simulink model ""  (R2019b)
settings: Solver=VariableStepAuto  StartTime=0.0  StopTime=200  RelTol=1e-3
model workspace (MAT data in the model file):
  x2xx = 0
values from neighbouring files (symbols this model uses):
  KDspd = 0    [frequency_validation.m]
  KIspd = 0    [frequency_validation.m]
  KPspd = 20    [frequency_validation.m]
  PARSa = [ ... (first row only)    [Q_ART_par.m]
  PARSu = zeros(Nu,5)    [Q_ART_par.m]
  Q0 = zeros(Nu+2,1)    [frequency_validation.m]
  QD0 = Q0    [frequency_validation.m]
  v_ref = vconst    (= 5.55555555556)    [frequency_validation.m]
undefined symbols (not defined in the file or in its folder): axle_rate_limit, Lspd, Nspd, Tmc, Uspd
libraries: simulink x2
(part 1 of 3)
settings Model: Creator=DJW  LastModifiedBy=14668

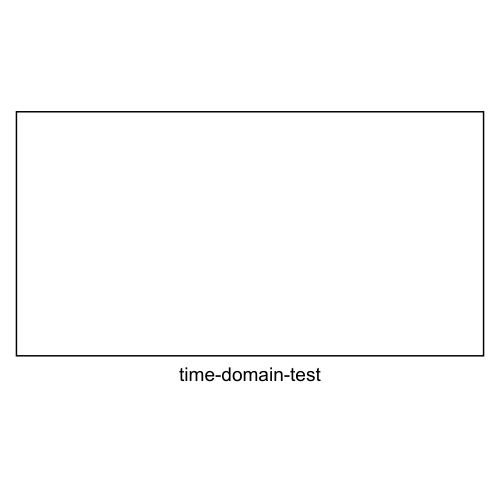
[thumbnail: Simulink's stored preview of the top-level diagram]
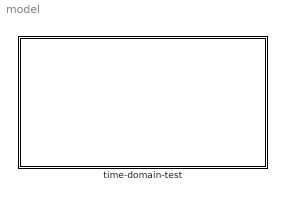
== system model ==
  time-domain-test : Subsystem

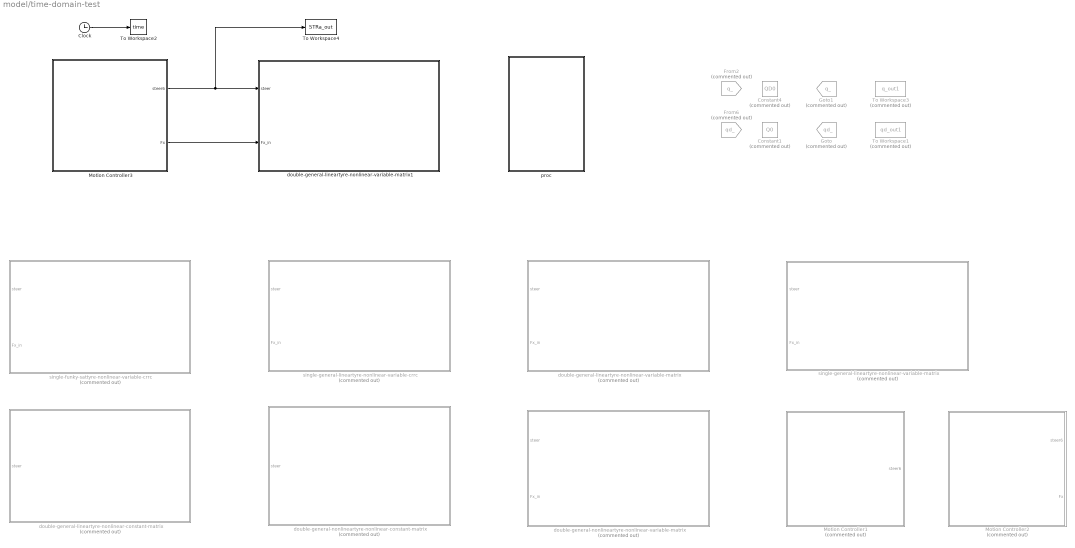
== system model/time-domain-test ==
  " Motion Controller1" : Subsystem  Commented=on  SystemSampleTime=Tmc
  " Motion Controller2" : Subsystem  Commented=on  SystemSampleTime=Tmc
  " Motion Controller3" : Subsystem  SystemSampleTime=Tmc
  Clock : Clock
  Constant1 : Constant  Commented=on  Value=Q0
  Constant4 : Constant  Commented=on  Value=QD0
  From2 : From  Commented=on  GotoTag=q_  TagVisibility=global
  From6 : From  Commented=on  GotoTag=qd_  TagVisibility=global
  Goto : Goto  Commented=on  GotoTag=qd_  TagVisibility=global
  Goto1 : Goto  Commented=on  GotoTag=q_  TagVisibility=global
  To Workspace1 : ToWorkspace  Commented=on  VariableName=qd_out1  SampleTime=-1
  To Workspace2 : ToWorkspace  VariableName=time  SampleTime=-1
  To Workspace3 : ToWorkspace  Commented=on  VariableName=q_out1  SampleTime=-1
  To Workspace4 : ToWorkspace  VariableName=STRa_out  SampleTime=-1
  double-general-lineartyre-nonlinear-constant-matrix : Subsystem  Commented=on
  double-general-lineartyre-nonlinear-variable-matrix : Subsystem  Commented=on
  double-general-lineartyre-nonlinear-variable-matrix1 : Subsystem
  double-general-nonlineartyre-nonlinear-constant-matrix : Subsystem  Commented=on
  double-general-nonlineartyre-nonlinear-variable-matrix : Subsystem  Commented=on
  proc : Subsystem
  single-funky-sattyre-nonlinear-variable-crrc : Subsystem  Commented=on
  single-general-lineartyre-nonlinear-variable-crrc : Subsystem  Commented=on
  single-general-lineartyre-nonlinear-variable-matrix : Subsystem  Commented=on
  wires:
  Clock/1 -> To Workspace2/1
  " Motion Controller3"/1(steer6) -> To Workspace4/1, double-general-lineartyre-nonlinear-variable-matrix1/1(steer)
  " Motion Controller3"/2(Fx) -> double-general-lineartyre-nonlinear-variable-matrix1/2(Fx_in)

== system model/time-domain-test/ Motion Controller1 ==
  Rate Transition6 : RateTransition
  discrete-time subsystem : Subsystem  TreatAsAtomicUnit=on  SystemSampleTime=Tmc
  steer6 : Outport
  wires:
  Rate Transition6/1 -> steer6/1
  discrete-time subsystem/1(steer) -> Rate Transition6/1

== system model/time-domain-test/ Motion Controller2 ==
  Rate Transition{3..6} (4 alike) : RateTransition
  discrete-time subsystem : Subsystem  TreatAsAtomicUnit=on  SystemSampleTime=Tmc
  steer6 : Outport
  Fx : Outport  Port=2
  wires:
  [q_] -> Rate Transition4/1
  Rate Transition5/1 -> Fx/1
  Rate Transition6/1 -> steer6/1
  [qd_] -> Rate Transition3/1
  discrete-time subsystem/1(steer) -> Rate Transition6/1
  Rate Transition4/1 -> discrete-time subsystem/1(q_in)
  Rate Transition3/1 -> discrete-time subsystem/2(qd_in)
  discrete-time subsystem/2(Fx_input) -> Rate Transition5/1

== system model/time-domain-test/ Motion Controller3 ==
  Rate Transition{3..6} (4 alike) : RateTransition
  discrete-time subsystem : Subsystem  TreatAsAtomicUnit=on  SystemSampleTime=Tmc
  steer6 : Outport
  Fx : Outport  Port=2
  wires:
  [q_] -> Rate Transition4/1
  Rate Transition5/1 -> Fx/1
  Rate Transition6/1 -> steer6/1
  [qd_] -> Rate Transition3/1
  discrete-time subsystem/1(steer) -> Rate Transition6/1
  Rate Transition4/1 -> discrete-time subsystem/1(q_in)
  Rate Transition3/1 -> discrete-time subsystem/2(qd_in)
  discrete-time subsystem/2(Fx_input) -> Rate Transition5/1

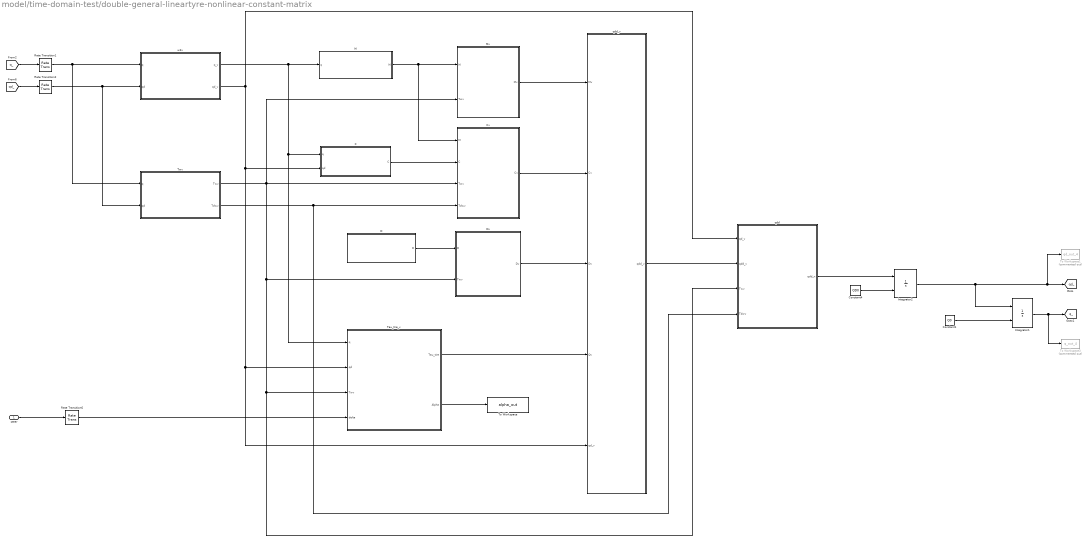
== system model/time-domain-test/double-general-lineartyre-nonlinear-constant-matrix ==
  steer : Inport
  C : MATLAB Function  TreatAsAtomicUnit=on
  Constant1 : Constant  Value=Q0
  Constant4 : Constant  Value=QD0
  Cv : MATLAB Function  TreatAsAtomicUnit=on
  D : MATLAB Function  TreatAsAtomicUnit=on
  Dv : MATLAB Function  TreatAsAtomicUnit=on
  Integrator1 : Integrator  InitialConditionSource=external  InitialCondition=Q0
  Integrator2 : Integrator  InitialConditionSource=external  InitialCondition=zeros(5,1)
  M : MATLAB Function  TreatAsAtomicUnit=on
  Mv : MATLAB Function  TreatAsAtomicUnit=on
  Rate Transition1 : RateTransition
  Rate Transition2 : RateTransition
  Rate Transition6 : RateTransition
  Tau_tire_v : MATLAB Function  TreatAsAtomicUnit=on
  To Workspace : ToWorkspace  VariableName=alpha_out  SampleTime=-1
  To Workspace1 : ToWorkspace  Commented=on  VariableName=qd_out_4  SampleTime=-1
  To Workspace3 : ToWorkspace  Commented=on  VariableName=q_out_4  SampleTime=-1
  Twv : MATLAB Function  TreatAsAtomicUnit=on
  qdd : MATLAB Function  TreatAsAtomicUnit=on
  qdd_v : MATLAB Function  TreatAsAtomicUnit=on
  w2v : MATLAB Function  TreatAsAtomicUnit=on
  tag scope: q_=global, qd_=global
  wires:
  M/1(M) -> Cv/1(M), Mv/1(M)
  [q_] -> Rate Transition1/1
  [qd_] -> Rate Transition2/1
  Twv/1(Twv) -> qdd/3(Twv), Tau_tire_v/3(Twv), Dv/2(Twv), Cv/3(Twv), Mv/2(Twv)
  C/1(C) -> Cv/2(C)
  Twv/2(Tdwv) -> qdd/4(Tdwv), Cv/4(Tdwv)
  D/1(D) -> Dv/1(D)
  steer/1 -> Rate Transition6/1
  w2v/1(q_v) -> M/1(q), Tau_tire_v/1(q), C/1(q)
  Mv/1(Mv) -> qdd_v/1(Mv)
  Dv/1(Dv) -> qdd_v/3(Dv)
  Cv/1(Cv) -> qdd_v/2(Cv)
  Tau_tire_v/1(Tau_tire) -> qdd_v/4(Qv)
  w2v/2(qd_v) -> qdd/1(qd_v), Tau_tire_v/2(qd), qdd_v/5(qd_v), C/2(qd)
  qdd_v/1(qdd_v) -> qdd/2(qdd_v)
  qdd/1(qdd_n) -> Integrator2/1
  Integrator1/1 -> To Workspace3/1, [q_]
  Integrator2/1 -> To Workspace1/1, [qd_], Integrator1/1
  Tau_tire_v/2(Alpha) -> To Workspace/1
  Constant4/1 -> Integrator2/2
  Constant1/1 -> Integrator1/2
  Rate Transition6/1 -> Tau_tire_v/4(delta)
  Rate Transition1/1 -> Twv/1(q), w2v/1(q)
  Rate Transition2/1 -> Twv/2(qd), w2v/2(qd)

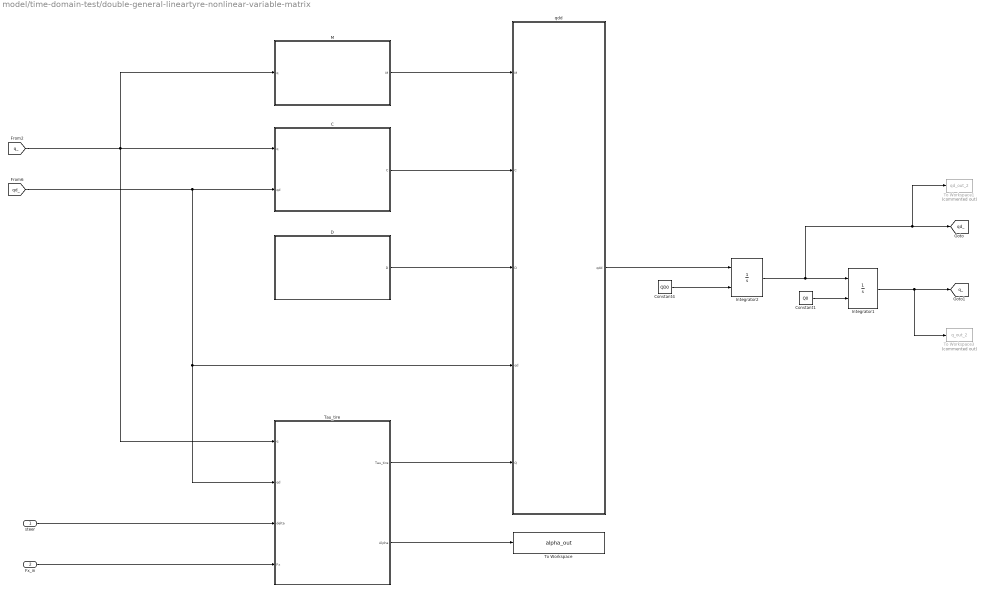
== system model/time-domain-test/double-general-lineartyre-nonlinear-variable-matrix ==
  steer : Inport
  Fx_in : Inport  Port=2
  C : MATLAB Function  TreatAsAtomicUnit=on
  Constant1 : Constant  Value=Q0
  Constant4 : Constant  Value=QD0
  D : MATLAB Function  TreatAsAtomicUnit=on
  Integrator1 : Integrator  InitialConditionSource=external  InitialCondition=Q0
  Integrator2 : Integrator  InitialConditionSource=external  InitialCondition=zeros(5,1)
  M : MATLAB Function  TreatAsAtomicUnit=on
  Tau_tire : MATLAB Function  TreatAsAtomicUnit=on
  To Workspace : ToWorkspace  VariableName=alpha_out  SampleTime=-1
  To Workspace1 : ToWorkspace  Commented=on  VariableName=qd_out_2  SampleTime=-1
  To Workspace3 : ToWorkspace  Commented=on  VariableName=q_out_2  SampleTime=-1
  qdd : MATLAB Function  TreatAsAtomicUnit=on
  tag scope: q_=global, qd_=global
  wires:
  Integrator1/1 -> To Workspace3/1, [q_]
  Fx_in/1 -> Tau_tire/4(Fx)
  [q_] -> Tau_tire/1(q), M/1(q), C/1(q)
  [qd_] -> Tau_tire/2(qd), qdd/4(qd), C/2(qd)
  steer/1 -> Tau_tire/3(delta)
  Tau_tire/2(Alpha) -> To Workspace/1
  qdd/1(qdd) -> Integrator2/1
  Integrator2/1 -> To Workspace1/1, [qd_], Integrator1/1
  M/1(M) -> qdd/1(M)
  C/1(C) -> qdd/2(C)
  Tau_tire/1(Tau_tire) -> qdd/5(Q)
  D/1(D) -> qdd/3(D)
  Constant4/1 -> Integrator2/2
  Constant1/1 -> Integrator1/2

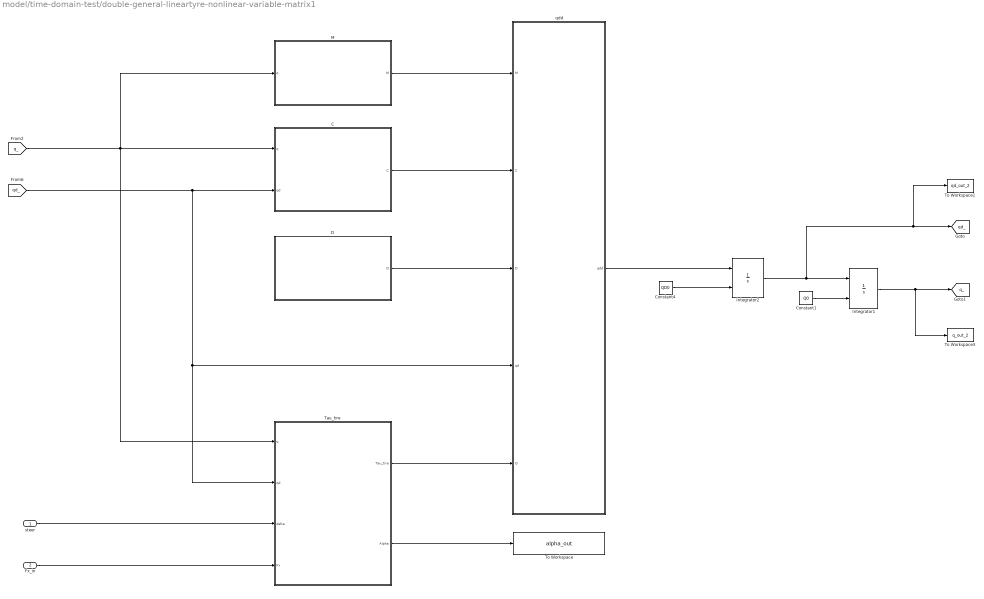
== system model/time-domain-test/double-general-lineartyre-nonlinear-variable-matrix1 ==
  steer : Inport
  Fx_in : Inport  Port=2
  C : MATLAB Function  TreatAsAtomicUnit=on
  Constant1 : Constant  Value=Q0
  Constant4 : Constant  Value=QD0
  D : MATLAB Function  TreatAsAtomicUnit=on
  Integrator1 : Integrator  InitialConditionSource=external  InitialCondition=Q0
  Integrator2 : Integrator  InitialConditionSource=external  InitialCondition=zeros(5,1)
  M : MATLAB Function  TreatAsAtomicUnit=on
  Tau_tire : MATLAB Function  TreatAsAtomicUnit=on
  To Workspace : ToWorkspace  VariableName=alpha_out  SampleTime=-1
  To Workspace1 : ToWorkspace  VariableName=qd_out_2  SampleTime=-1
  To Workspace3 : ToWorkspace  VariableName=q_out_2  SampleTime=-1
  qdd : MATLAB Function  TreatAsAtomicUnit=on
  tag scope: q_=global, qd_=global
  wires:
  Integrator1/1 -> To Workspace3/1, [q_]
  Fx_in/1 -> Tau_tire/4(Fx)
  [q_] -> Tau_tire/1(q), M/1(q), C/1(q)
  [qd_] -> Tau_tire/2(qd), qdd/4(qd), C/2(qd)
  steer/1 -> Tau_tire/3(delta)
  Tau_tire/2(Alpha) -> To Workspace/1
  qdd/1(qdd) -> Integrator2/1
  Integrator2/1 -> To Workspace1/1, [qd_], Integrator1/1
  M/1(M) -> qdd/1(M)
  C/1(C) -> qdd/2(C)
  Tau_tire/1(Tau_tire) -> qdd/5(Q)
  D/1(D) -> qdd/3(D)
  Constant4/1 -> Integrator2/2
  Constant1/1 -> Integrator1/2

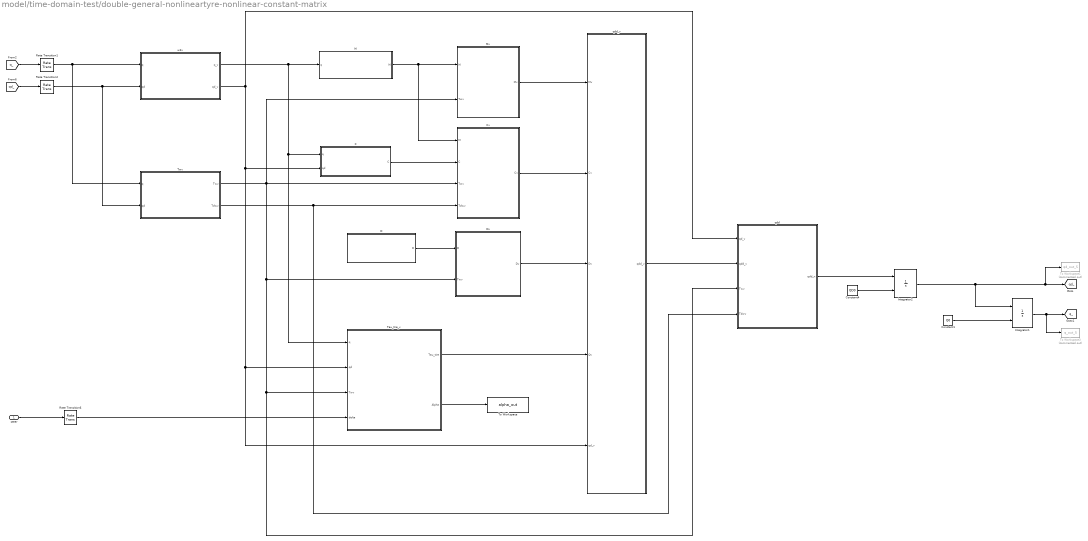
== system model/time-domain-test/double-general-nonlineartyre-nonlinear-constant-matrix ==
  steer : Inport
  C : MATLAB Function  TreatAsAtomicUnit=on
  Constant1 : Constant  Value=Q0
  Constant4 : Constant  Value=QD0
  Cv : MATLAB Function  TreatAsAtomicUnit=on
  D : MATLAB Function  TreatAsAtomicUnit=on
  Dv : MATLAB Function  TreatAsAtomicUnit=on
  Integrator1 : Integrator  InitialConditionSource=external  InitialCondition=Q0
  Integrator2 : Integrator  InitialConditionSource=external  InitialCondition=zeros(5,1)
  M : MATLAB Function  TreatAsAtomicUnit=on
  Mv : MATLAB Function  TreatAsAtomicUnit=on
  Rate Transition1 : RateTransition
  Rate Transition2 : RateTransition
  Rate Transition6 : RateTransition
  Tau_tire_v : MATLAB Function  TreatAsAtomicUnit=on
  To Workspace : ToWorkspace  VariableName=alpha_out  SampleTime=-1
  To Workspace1 : ToWorkspace  Commented=on  VariableName=qd_out_5  SampleTime=-1
  To Workspace3 : ToWorkspace  Commented=on  VariableName=q_out_5  SampleTime=-1
  Twv : MATLAB Function  TreatAsAtomicUnit=on
  qdd : MATLAB Function  TreatAsAtomicUnit=on
  qdd_v : MATLAB Function  TreatAsAtomicUnit=on
  w2v : MATLAB Function  TreatAsAtomicUnit=on
  tag scope: q_=global, qd_=global
  wires:
  M/1(M) -> Cv/1(M), Mv/1(M)
  [q_] -> Rate Transition1/1
  [qd_] -> Rate Transition2/1
  Twv/1(Twv) -> qdd/3(Twv), Tau_tire_v/3(Twv), Dv/2(Twv), Cv/3(Twv), Mv/2(Twv)
  C/1(C) -> Cv/2(C)
  Twv/2(Tdwv) -> qdd/4(Tdwv), Cv/4(Tdwv)
  D/1(D) -> Dv/1(D)
  steer/1 -> Rate Transition6/1
  w2v/1(q_v) -> M/1(q), Tau_tire_v/1(q), C/1(q)
  Mv/1(Mv) -> qdd_v/1(Mv)
  Dv/1(Dv) -> qdd_v/3(Dv)
  Cv/1(Cv) -> qdd_v/2(Cv)
  Tau_tire_v/1(Tau_tire) -> qdd_v/4(Qv)
  w2v/2(qd_v) -> qdd/1(qd_v), Tau_tire_v/2(qd), qdd_v/5(qd_v), C/2(qd)
  qdd_v/1(qdd_v) -> qdd/2(qdd_v)
  qdd/1(qdd_n) -> Integrator2/1
  Integrator1/1 -> To Workspace3/1, [q_]
  Integrator2/1 -> To Workspace1/1, [qd_], Integrator1/1
  Tau_tire_v/2(Alpha) -> To Workspace/1
  Constant4/1 -> Integrator2/2
  Constant1/1 -> Integrator1/2
  Rate Transition6/1 -> Tau_tire_v/4(delta)
  Rate Transition1/1 -> Twv/1(q), w2v/1(q)
  Rate Transition2/1 -> Twv/2(qd), w2v/2(qd)

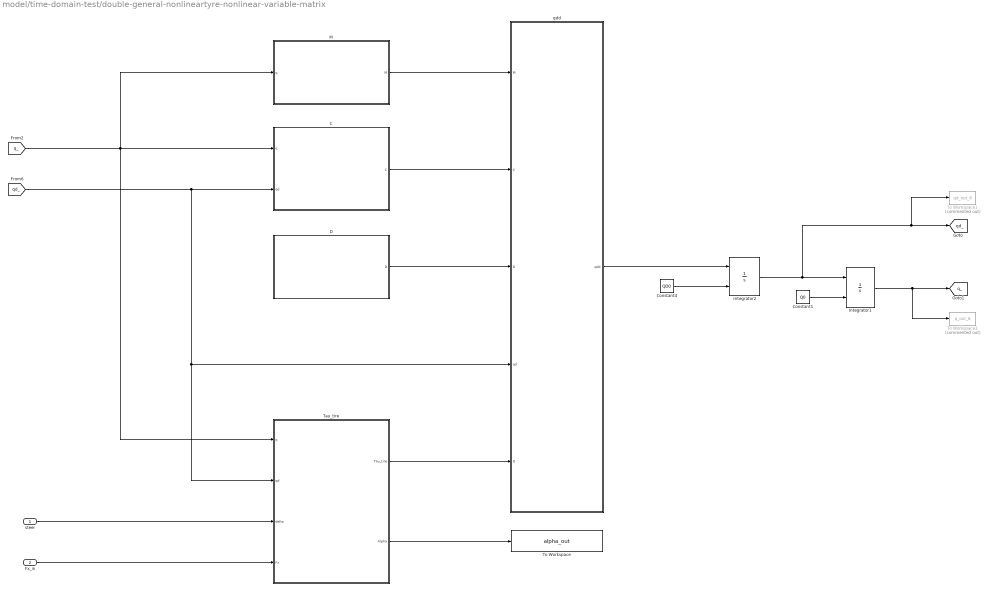
== system model/time-domain-test/double-general-nonlineartyre-nonlinear-variable-matrix ==
  steer : Inport
  Fx_in : Inport  Port=2
  C : MATLAB Function  TreatAsAtomicUnit=on
  Constant1 : Constant  Value=Q0
  Constant4 : Constant  Value=QD0
  D : MATLAB Function  TreatAsAtomicUnit=on
  Integrator1 : Integrator  InitialConditionSource=external  InitialCondition=Q0
  Integrator2 : Integrator  InitialConditionSource=external  InitialCondition=zeros(5,1)
  M : MATLAB Function  TreatAsAtomicUnit=on
  Tau_tire : MATLAB Function  TreatAsAtomicUnit=on
  To Workspace : ToWorkspace  VariableName=alpha_out  SampleTime=-1
  To Workspace1 : ToWorkspace  Commented=on  VariableName=qd_out_6  SampleTime=-1
  To Workspace3 : ToWorkspace  Commented=on  VariableName=q_out_6  SampleTime=-1
  qdd : MATLAB Function  TreatAsAtomicUnit=on
  tag scope: q_=global, qd_=global
  wires:
  Integrator1/1 -> To Workspace3/1, [q_]
  Fx_in/1 -> Tau_tire/4(Fx)
  [q_] -> Tau_tire/1(q), M/1(q), C/1(q)
  [qd_] -> Tau_tire/2(qd), qdd/4(qd), C/2(qd)
  steer/1 -> Tau_tire/3(delta)
  Tau_tire/2(Alpha) -> To Workspace/1
  qdd/1(qdd) -> Integrator2/1
  Integrator2/1 -> To Workspace1/1, [qd_], Integrator1/1
  M/1(M) -> qdd/1(M)
  C/1(C) -> qdd/2(C)
  Tau_tire/1(Tau_tire) -> qdd/5(Q)
  D/1(D) -> qdd/3(D)
  Constant4/1 -> Integrator2/2
  Constant1/1 -> Integrator1/2

== system model/time-domain-test/proc ==
  Constant1 : Constant  Value=PARSu
  Constant2 : Constant  Value=PARSa
  MatMaker : MATLAB Function  TreatAsAtomicUnit=on
  To Workspace1 : ToWorkspace  VariableName=Va_out  SampleTime=-1
  To Workspace3 : ToWorkspace  VariableName=Vj_out  SampleTime=-1
  To Workspace5 : ToWorkspace  VariableName=Vg_out  SampleTime=-1
  To Workspace6 : ToWorkspace  VariableName=Vgg_out  SampleTime=-1
  To Workspace7 : ToWorkspace  VariableName=Vaa_out  SampleTime=-1
  wires:
  [qd_] -> MatMaker/2(qd)
  MatMaker/1(Va) -> To Workspace1/1
  [q_] -> MatMaker/1(q)
  MatMaker/5(Vgg) -> To Workspace6/1
  MatMaker/3(Vj) -> To Workspace3/1
  Constant1/1 -> MatMaker/3(PARSu)
  MatMaker/4(Vg) -> To Workspace5/1
  Constant2/1 -> MatMaker/4(PARSa)
  MatMaker/2(Vaa) -> To Workspace7/1

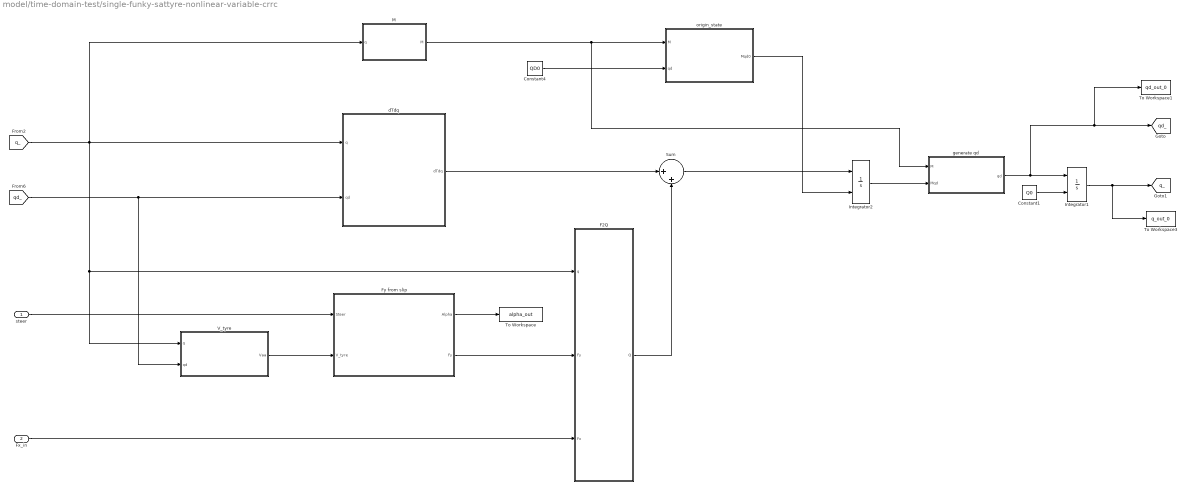
== system model/time-domain-test/single-funky-sattyre-nonlinear-variable-crrc ==
  steer : Inport
  Fx_in : Inport  Port=2
  Constant1 : Constant  Value=Q0
  Constant4 : Constant  Value=QD0
  F2Q : MATLAB Function  TreatAsAtomicUnit=on
  Fy from slip : MATLAB Function  TreatAsAtomicUnit=on
  Integrator1 : Integrator  InitialConditionSource=external  InitialCondition=Q0
  Integrator2 : Integrator  InitialConditionSource=external  InitialCondition=QD0
  M : MATLAB Function  TreatAsAtomicUnit=on
  Sum : Sum  Inputs=|++
  To Workspace : ToWorkspace  VariableName=alpha_out  SampleTime=-1
  To Workspace1 : ToWorkspace  VariableName=qd_out_0  SampleTime=-1
  To Workspace3 : ToWorkspace  VariableName=q_out_0  SampleTime=-1
  V_tyre : MATLAB Function  TreatAsAtomicUnit=on
  dTdq : MATLAB Function  TreatAsAtomicUnit=on
  generate qd : MATLAB Function  TreatAsAtomicUnit=on
  origin_state : MATLAB Function  TreatAsAtomicUnit=on
  tag scope: q_=global, qd_=global
  wires:
  Fy from slip/2(Fy) -> F2Q/2(Fy)
  Integrator1/1 -> To Workspace3/1, [q_]
  Fx_in/1 -> F2Q/3(Fx)
  dTdq/1(dTdq) -> Sum/1
  steer/1 -> Fy from slip/1(Steer)
  F2Q/1(Q) -> Sum/2
  V_tyre/1(Vaa) -> Fy from slip/2(V_tyre)
  Sum/1 -> Integrator2/1
  origin_state/1(Mqd0) -> Integrator2/2
  M/1(M) -> generate qd/1(M), origin_state/1(M)
  Integrator2/1 -> generate qd/2(Mqd)
  [q_] -> dTdq/1(q), V_tyre/1(q), F2Q/1(q), M/1(q)
  [qd_] -> dTdq/2(qd), V_tyre/2(qd)
  Fy from slip/1(Alpha) -> To Workspace/1
  Constant4/1 -> origin_state/2(qd)
  Constant1/1 -> Integrator1/2
  generate qd/1(qd) -> To Workspace1/1, [qd_], Integrator1/1

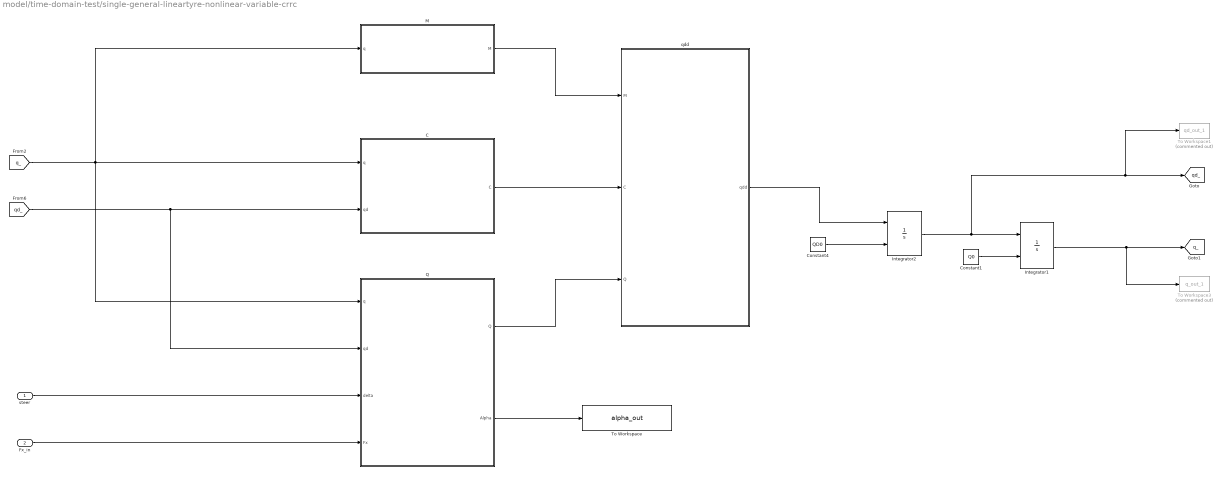
== system model/time-domain-test/single-general-lineartyre-nonlinear-variable-crrc ==
  steer : Inport
  Fx_in : Inport  Port=2
  C : MATLAB Function  TreatAsAtomicUnit=on
  Constant1 : Constant  Value=Q0
  Constant4 : Constant  Value=QD0
  Integrator1 : Integrator  InitialConditionSource=external  InitialCondition=Q0
  Integrator2 : Integrator  InitialConditionSource=external  InitialCondition=zeros(5,1)
  M : MATLAB Function  TreatAsAtomicUnit=on
  Q : MATLAB Function  TreatAsAtomicUnit=on
  To Workspace : ToWorkspace  VariableName=alpha_out  SampleTime=-1
  To Workspace1 : ToWorkspace  Commented=on  VariableName=qd_out_1  SampleTime=-1
  To Workspace3 : ToWorkspace  Commented=on  VariableName=q_out_1  SampleTime=-1
  qdd : MATLAB Function  TreatAsAtomicUnit=on
  tag scope: q_=global, qd_=global
  wires:
  Integrator1/1 -> To Workspace3/1, [q_]
  Fx_in/1 -> Q/4(Fx)
  [q_] -> M/1(q), C/1(q), Q/1(q)
  [qd_] -> Q/2(qd), C/2(qd)
  steer/1 -> Q/3(delta)
  Q/2(Alpha) -> To Workspace/1
  qdd/1(qdd) -> Integrator2/1
  Integrator2/1 -> To Workspace1/1, [qd_], Integrator1/1
  M/1(M) -> qdd/1(M)
  C/1(C) -> qdd/2(C)
  Q/1(Q) -> qdd/3(Q)
  Constant4/1 -> Integrator2/2
  Constant1/1 -> Integrator1/2

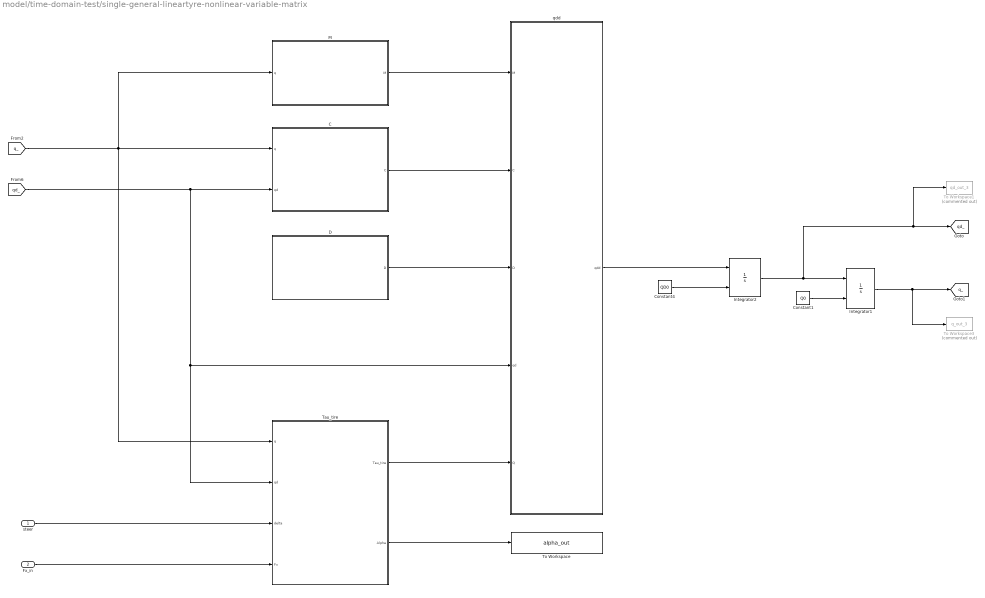
== system model/time-domain-test/single-general-lineartyre-nonlinear-variable-matrix ==
  steer : Inport
  Fx_in : Inport  Port=2
  C : MATLAB Function  TreatAsAtomicUnit=on
  Constant1 : Constant  Value=Q0
  Constant4 : Constant  Value=QD0
  D : MATLAB Function  TreatAsAtomicUnit=on
  Integrator1 : Integrator  InitialConditionSource=external  InitialCondition=Q0
  Integrator2 : Integrator  InitialConditionSource=external  InitialCondition=zeros(5,1)
  M : MATLAB Function  TreatAsAtomicUnit=on
  Tau_tire : MATLAB Function  TreatAsAtomicUnit=on
  To Workspace : ToWorkspace  VariableName=alpha_out  SampleTime=-1
  To Workspace1 : ToWorkspace  Commented=on  VariableName=qd_out_3  SampleTime=-1
  To Workspace3 : ToWorkspace  Commented=on  VariableName=q_out_3  SampleTime=-1
  qdd : MATLAB Function  TreatAsAtomicUnit=on
  tag scope: q_=global, qd_=global
  wires:
  Integrator1/1 -> To Workspace3/1, [q_]
  Fx_in/1 -> Tau_tire/4(Fx)
  [q_] -> Tau_tire/1(q), M/1(q), C/1(q)
  [qd_] -> Tau_tire/2(qd), qdd/4(qd), C/2(qd)
  steer/1 -> Tau_tire/3(delta)
  Tau_tire/2(Alpha) -> To Workspace/1
  qdd/1(qdd) -> Integrator2/1
  M/1(M) -> qdd/1(M)
  C/1(C) -> qdd/2(C)
  Tau_tire/1(Tau_tire) -> qdd/5(Q)
  D/1(D) -> qdd/3(D)
  Constant4/1 -> Integrator2/2
  Constant1/1 -> Integrator1/2
  Integrator2/1 -> To Workspace1/1, [qd_], Integrator1/1

== system model/time-domain-test/ Motion Controller1/discrete-time subsystem ==
  note: steering ratio
  note: OL steering wheel angle in rad
  Constant3 : Constant  Value=PARSa
  Digital Clock1 : DigitalClock  SampleTime=-1
  From Workspace : FromWorkspace  VariableName=[tstr_in,str_in]  SampleTime=-1
  Gain1 : Gain  Gain=1/20
  MATLAB Function : MATLAB Function  TreatAsAtomicUnit=on
  Rate Limiter1 : RateLimiter  RisingSlewLimit=axle_rate_limit  FallingSlewLimit=-axle_rate_limit  SampleTimeMode=inherited
  To Workspace3 : ToWorkspace  VariableName=tdig_out1  SampleTime=-1
  steer : Outport
  wires:
  Digital Clock1/1 -> To Workspace3/1
  From Workspace/1 -> Gain1/1
  Gain1/1 -> MATLAB Function/1(str1)
  MATLAB Function/1(y) -> Rate Limiter1/1
  Constant3/1 -> MATLAB Function/2(PARSa)
  Rate Limiter1/1 -> steer/1

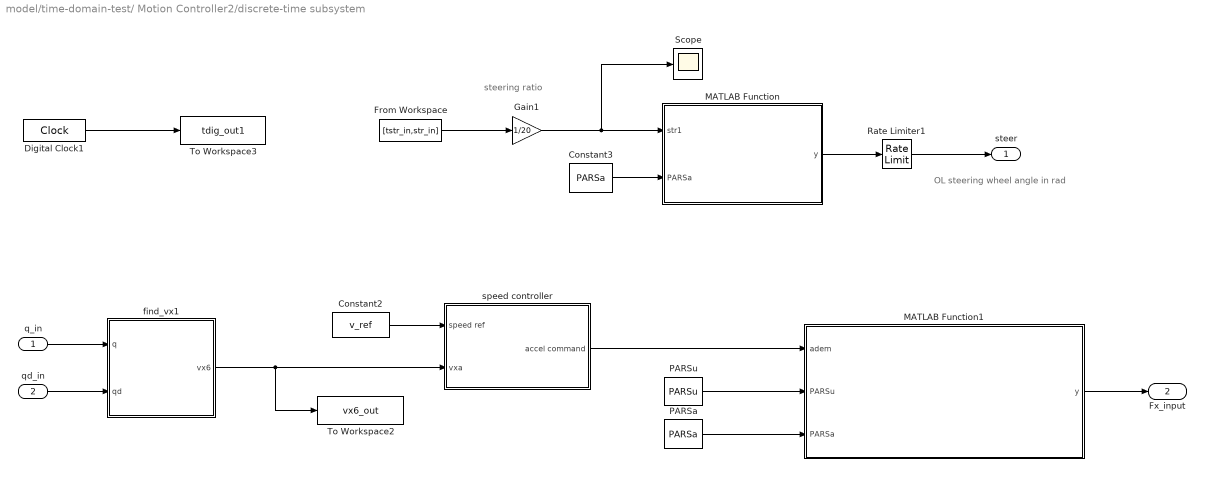
== system model/time-domain-test/ Motion Controller2/discrete-time subsystem ==
  note: steering ratio
  note: OL steering wheel angle in rad
  q_in : Inport
  qd_in : Inport  Port=2
  " PARSu" : Constant  Value=PARSu
  Constant2 : Constant  Value=v_ref
  Constant3 : Constant  Value=PARSa
  Digital Clock1 : DigitalClock  SampleTime=-1
  From Workspace : FromWorkspace  VariableName=[tstr_in,str_in]  SampleTime=-1
  Gain1 : Gain  Gain=1/20
  MATLAB Function : MATLAB Function  TreatAsAtomicUnit=on
  MATLAB Function1 : MATLAB Function  TreatAsAtomicUnit=on
  PARSa : Constant  Value=PARSa
  Rate Limiter1 : RateLimiter  RisingSlewLimit=axle_rate_limit  FallingSlewLimit=-axle_rate_limit  SampleTimeMode=inherited
  Scope : Scope
  To Workspace2 : ToWorkspace  VariableName=vx6_out  SampleTime=-1
  To Workspace3 : ToWorkspace  VariableName=tdig_out1  SampleTime=-1
  find_vx1 : MATLAB Function  TreatAsAtomicUnit=on
  speed controller : Subsystem
  steer : Outport
  Fx_input : Outport  Port=2  VectorParamsAs1DForOutWhenUnconnected=off
  wires:
  q_in/1 -> find_vx1/1(q)
  Constant2/1 -> speed controller/1(speed ref)
  qd_in/1 -> find_vx1/2(qd)
  find_vx1/1(vx6) -> speed controller/2(vxa), To Workspace2/1
  Digital Clock1/1 -> To Workspace3/1
  From Workspace/1 -> Gain1/1
  Gain1/1 -> Scope/1, MATLAB Function/1(str1)
  MATLAB Function/1(y) -> Rate Limiter1/1
  Constant3/1 -> MATLAB Function/2(PARSa)
  Rate Limiter1/1 -> steer/1
  MATLAB Function1/1(y) -> Fx_input/1
  " PARSu"/1 -> MATLAB Function1/2(PARSu)
  PARSa/1 -> MATLAB Function1/3(PARSa)
  speed controller/1(accel command) -> MATLAB Function1/1(adem)

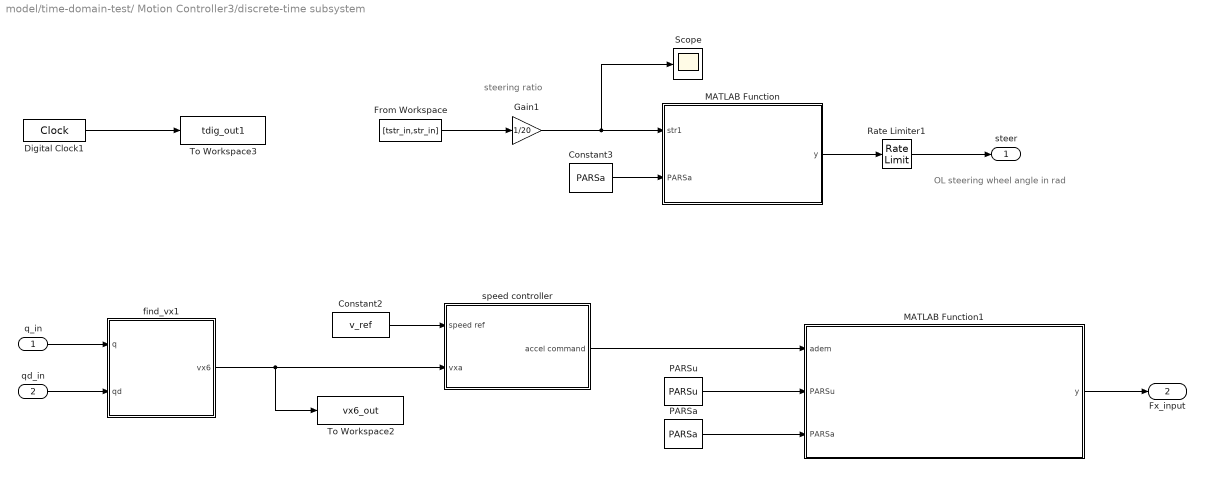
== system model/time-domain-test/ Motion Controller3/discrete-time subsystem ==
  note: steering ratio
  note: OL steering wheel angle in rad
  q_in : Inport
  qd_in : Inport  Port=2
  " PARSu" : Constant  Value=PARSu
  Constant2 : Constant  Value=v_ref
  Constant3 : Constant  Value=PARSa
  Digital Clock1 : DigitalClock  SampleTime=-1
  From Workspace : FromWorkspace  VariableName=[tstr_in,str_in]  SampleTime=-1
  Gain1 : Gain  Gain=1/20
  MATLAB Function : MATLAB Function  TreatAsAtomicUnit=on
  MATLAB Function1 : MATLAB Function  TreatAsAtomicUnit=on
  PARSa : Constant  Value=PARSa
  Rate Limiter1 : RateLimiter  RisingSlewLimit=axle_rate_limit  FallingSlewLimit=-axle_rate_limit  SampleTimeMode=inherited
  Scope : Scope
  To Workspace2 : ToWorkspace  VariableName=vx6_out  SampleTime=-1
  To Workspace3 : ToWorkspace  VariableName=tdig_out1  SampleTime=-1
  find_vx1 : MATLAB Function  TreatAsAtomicUnit=on
  speed controller : Subsystem
  steer : Outport
  Fx_input : Outport  Port=2  VectorParamsAs1DForOutWhenUnconnected=off
  wires:
  q_in/1 -> find_vx1/1(q)
  Constant2/1 -> speed controller/1(speed ref)
  qd_in/1 -> find_vx1/2(qd)
  find_vx1/1(vx6) -> speed controller/2(vxa), To Workspace2/1
  Digital Clock1/1 -> To Workspace3/1
  From Workspace/1 -> Gain1/1
  Gain1/1 -> Scope/1, MATLAB Function/1(str1)
  MATLAB Function/1(y) -> Rate Limiter1/1
  Constant3/1 -> MATLAB Function/2(PARSa)
  Rate Limiter1/1 -> steer/1
  MATLAB Function1/1(y) -> Fx_input/1
  " PARSu"/1 -> MATLAB Function1/2(PARSu)
  PARSa/1 -> MATLAB Function1/3(PARSa)
  speed controller/1(accel command) -> MATLAB Function1/1(adem)

== system model/time-domain-test/ Motion Controller2/discrete-time subsystem/speed controller ==
  speed ref : Inport
  vxa : Inport  Port=2
  PID Controller : simulink/Continuous/PID Controller  Controller=PID  Form=Parallel  TimeDomain=Discrete-time  SampleTime=-1  IntegratorMethod=Forward Euler  FilterMethod=Forward Euler  ControllerParametersSource=internal  P=KPspd  I=KIspd  D=KDspd  N=Nspd  UseFilter=on  TunerSelectOption=Transfer Function Based (PID Tuner App)  InitialConditionSource=internal  InitialConditionForIntegrator=0  InitialConditionForFilter=0  DifferentiatorICPrevScaledInput=0  ExternalReset=none  TrackingMode=off  Kt=1  LimitOutput=on  UpperSaturationLimit=Uspd  LowerSaturationLimit=Lspd  LinearizeAsGain=on  AntiWindupMode=clamping  Kb=1  POutMin=[]  POutMax=[]  IOutMin=[]  IOutMax=[]  DOutMin=[]  DOutMax=[]  NOutMin=[]  NOutMax=[]  SumOutMin=[]  SumOutMax=[]  SaturationOutMin=[]  SaturationOutMax=[]  PParamMin=[]  PParamMax=[]  IParamMin=[]  IParamMax=[]  DParamMin=[]  DParamMax=[]  NParamMin=[]  NParamMax=[]  KbParamMin=[]  KbParamMax=[]  KtParamMin=[]  KtParamMax=[]  KbOutMin=[]  KbOutMax=[]  KtOutMin=[]  KtOutMax=[]  IntegratorOutMin=[]  IntegratorOutMax=[]  FilterOutMin=[]  FilterOutMax=[]  SumI1OutMin=[]  SumI1OutMax=[]  SumI2OutMin=[]  SumI2OutMax=[]  SumI3OutMin=[]  SumI3OutMax=[]  SumI4OutMin=[]  SumI4OutMax=[]  SumDOutMin=[]  SumDOutMax=[]  DifferentiatorOutMin=[]  DifferentiatorOutMax=[]  FilterDiffOutCoefMin=[]  FilterDiffOutCoefMax=[]  ReciprocalOutMin=[]  ReciprocalOutMax=[]  SumDenOutMin=[]  SumDenOutMax=[]  SumNumOutMin=[]  SumNumOutMax=[]  DivideOutMin=[]  DivideOutMax=[]  IntegratorContinuousStateAttributes=''  IntegratorStateMustResolveToSignalObject=off  IntegratorRTWStateStorageClass=Auto  FilterContinuousStateAttributes=''  FilterStateMustResolveToSignalObject=off  FilterRTWStateStorageClass=Auto  ParallelPVariant=InternalParameters  IdealPVariant=Disabled  IVariant=InternalParameters  DVariant=InternalParameters  IntegratorVariant=Discrete  SatVariant=Enabled  AWVariant=DiscClampingParallel  PCopyVariant=Disabled  TRVariant=Disabled  FdbkBlocksVariant=Forward  IdealPFdbkVariant=Disabled  SatFdbkVariant=Disabled  DerivativeFilterVariant=ForwardEulerFilter  NVariant=InternalParameters  NCopyVariant=Disabled  FilterICVariant=InternalICsFilter  IntegratorICVariant=InternalICs  ExternalResetVariant=Disabled  TRSumVariant=Passthrough  SumFdbkVariant=Disabled  SumVariant=Sum_PID
  Sum : Sum  Inputs=|-+
  select U : Selector  InputPortWidth=6  IndexOptions=Index vector (dialog)  Indices=[1]  OutputSizes=1
  accel command : Outport
  wires:
  Sum/1 -> PID Controller/1
  vxa/1 -> select U/1
  select U/1 -> Sum/1
  speed ref/1 -> Sum/2
  PID Controller/1 -> accel command/1

== system model/time-domain-test/ Motion Controller3/discrete-time subsystem/speed controller ==
  speed ref : Inport
  vxa : Inport  Port=2
  PID Controller : simulink/Continuous/PID Controller  Controller=PID  Form=Parallel  TimeDomain=Discrete-time  SampleTime=-1  IntegratorMethod=Forward Euler  FilterMethod=Forward Euler  ControllerParametersSource=internal  P=KPspd  I=KIspd  D=KDspd  N=Nspd  UseFilter=on  TunerSelectOption=Transfer Function Based (PID Tuner App)  InitialConditionSource=internal  InitialConditionForIntegrator=0  InitialConditionForFilter=0  DifferentiatorICPrevScaledInput=0  ExternalReset=none  TrackingMode=off  Kt=1  LimitOutput=on  UpperSaturationLimit=Uspd  LowerSaturationLimit=Lspd  LinearizeAsGain=on  AntiWindupMode=clamping  Kb=1  POutMin=[]  POutMax=[]  IOutMin=[]  IOutMax=[]  DOutMin=[]  DOutMax=[]  NOutMin=[]  NOutMax=[]  SumOutMin=[]  SumOutMax=[]  SaturationOutMin=[]  SaturationOutMax=[]  PParamMin=[]  PParamMax=[]  IParamMin=[]  IParamMax=[]  DParamMin=[]  DParamMax=[]  NParamMin=[]  NParamMax=[]  KbParamMin=[]  KbParamMax=[]  KtParamMin=[]  KtParamMax=[]  KbOutMin=[]  KbOutMax=[]  KtOutMin=[]  KtOutMax=[]  IntegratorOutMin=[]  IntegratorOutMax=[]  FilterOutMin=[]  FilterOutMax=[]  SumI1OutMin=[]  SumI1OutMax=[]  SumI2OutMin=[]  SumI2OutMax=[]  SumI3OutMin=[]  SumI3OutMax=[]  SumI4OutMin=[]  SumI4OutMax=[]  SumDOutMin=[]  SumDOutMax=[]  DifferentiatorOutMin=[]  DifferentiatorOutMax=[]  FilterDiffOutCoefMin=[]  FilterDiffOutCoefMax=[]  ReciprocalOutMin=[]  ReciprocalOutMax=[]  SumDenOutMin=[]  SumDenOutMax=[]  SumNumOutMin=[]  SumNumOutMax=[]  DivideOutMin=[]  DivideOutMax=[]  IntegratorContinuousStateAttributes=''  IntegratorStateMustResolveToSignalObject=off  IntegratorRTWStateStorageClass=Auto  FilterContinuousStateAttributes=''  FilterStateMustResolveToSignalObject=off  FilterRTWStateStorageClass=Auto  ParallelPVariant=InternalParameters  IdealPVariant=Disabled  IVariant=InternalParameters  DVariant=InternalParameters  IntegratorVariant=Discrete  SatVariant=Enabled  AWVariant=DiscClampingParallel  PCopyVariant=Disabled  TRVariant=Disabled  FdbkBlocksVariant=Forward  IdealPFdbkVariant=Disabled  SatFdbkVariant=Disabled  DerivativeFilterVariant=ForwardEulerFilter  NVariant=InternalParameters  NCopyVariant=Disabled  FilterICVariant=InternalICsFilter  IntegratorICVariant=InternalICs  ExternalResetVariant=Disabled  TRSumVariant=Passthrough  SumFdbkVariant=Disabled  SumVariant=Sum_PID
  Sum : Sum  Inputs=|-+
  select U : Selector  InputPortWidth=6  IndexOptions=Index vector (dialog)  Indices=[1]  OutputSizes=1
  accel command : Outport
  wires:
  Sum/1 -> PID Controller/1
  vxa/1 -> select U/1
  select U/1 -> Sum/1
  speed ref/1 -> Sum/2
  PID Controller/1 -> accel command/1

== matlab function time-domain-test/ Motion Controller3/discrete-time subsystem/MATLAB Function ==
  data: str1 input; y output; PARSa input
function y = StrMux(str1,PARSa)
%distribute steering from driver (and auto steer in future versions)
y=PARSa(:,6);
y=y*str1;
end

== matlab function time-domain-test/ Motion Controller3/discrete-time subsystem/MATLAB Function1 ==
  data: adem input; y output; PARSu input; PARSa input
function y = wheel_force_distibution(adem,PARSu,PARSa)

y=zeros(8,1); 
mass=sum(PARSu(:,1));
Na=size(PARSa,1);
if adem>0
    y(1:Na)=PARSa(:,4); %drive axle distribution
else
    y(1:Na)=PARSa(:,5); %brake force distribution
end
n=sum(y);
y=y*mass*adem/n;
end

== matlab function time-domain-test/single-funky-sattyre-nonlinear-variable-crrc/F2Q ==
  data: q input; Fy input; Fx input; Q output
function Q = fcn(q, Fy, Fx)

%%%%%%%%%%%%%%%%%%%%%%%%%%%%%%%%%%%%%%%%%%%%%%%%%%%%%%%%%%%%%%%%%%%%%%%%%%
% Parameter given

LL = [11.4, 9.4, 11.4]';
XA = [8.9, 7.4, 1.5, 7.9, 1.5, 9.9, 4.0, 2.5]';
IU = [1, 1, 1, 2, 2, 3, 3, 3]';
%%%%%%%%%%%%%%%%%%%%%%%%%%%%%%%%%%%%%%%%%%%%%%%%%%%%%%%%%%%%%%%%%%%%%%%%%%
% specify dimensition of matrix in advance

Q = zeros(5,1);
%%%%%%%%%%%%%%%%%%%%%%%%%%%%%%%%%%%%%%%%%%%%%%%%%%%%%%%%%%%%%%%%%%%%%%%%%%
% Rotation matrix

uu = zeros(2, 3); 
nn = zeros(2, 3); 
for i = 1:3
    c = cos(q(i + 2));
    s = sin(q(i + 2)); 
    uu(:, i)=[c, s]';
    nn(:, i)=[-s, c]';
end
%%%%%%%%%%%%%%%%%%%%%%%%%%%%%%%%%%%%%%%%%%%%%%%%%%%%%%%%%%%%%%%%%%%%%%%%%%
% calculate Q matrix

temp = zeros(2,5);
temp(1, 1) = 1;
temp(2, 2) = 1;

for i = 1:8
    Fa = [Fx(i); Fy(i)];
    iu = IU(i); 
    u = uu(:, iu);
    n = nn(:, iu);
    P = temp; 

    for j = 1:iu
        if j < iu
            P(:, j + 2) = -LL(j) * nn(:, j);
        else
            P(:, j + 2) = -(LL(j) - XA(i)) * nn(:, j);
        end
    end
    Q = Q + P' * [u n] * Fa;
end
%%%%%%%%%%%%%%%%%%%%%%%%%%%%%%%%%%%%%%%%%%%%%%%%%%%%%%%%%%%%%%%%%%%%%%%%%%

== matlab function time-domain-test/ Motion Controller3/discrete-time subsystem/find_vx1 ==
  settings: updateMethod=DISCRETE
  data: vx6 output; q input; qd input
function vx6 = vx_conversion(q,qd)
%#codegen
% convert q and qd to vx6 needed for the driver model

xxp=2; %nominal point P of driver 
u1=[cos(q(3));sin(q(3))];n1=[-sin(q(3));cos(q(3))];
rp = q(1:2)-xxp*u1;

v00=qd(1:2); %global velocity at front joint
vp=v00-qd(3)*xxp*n1; %move to driver point
U=dot(vp,u1);V=dot(vp,n1); %components in body axes (unit 1)
vx6=[U;V;qd(3);rp;q(3)]; %standard format ... [U,V,r,x,y,psi]'
end

== matlab function time-domain-test/double-general-lineartyre-nonlinear-variable-matrix1/C ==
  data: q input; qd input; C output
function C = calculate_C(q, qd)

m1 = 11142;
m3 = 11142;
m2 = 7651; 
l_j1j2 = 11.4;
l_j2j3 = 9.4;
l_j1g1 = 5.862; 
l_j2g2 = 4.643; 
l_j3g3 = 5.538; 

psi1 = q(3);
psi2 = q(4);
psi3 = q(5);
xd = qd(1);
yd = qd(2);
psi1d = qd(3);
psi2d = qd(4);
psi3d = qd(5);

C = [0, 0, (l_j1g1*m1 + l_j1j2*(m2 + m3))*cos(psi1)*psi1d, (l_j2g2*m2 + l_j2j3*m3)*cos(psi2)*psi2d, l_j3g3*m3*cos(psi3)*psi3d;
     0, 0, (l_j1g1*m1 + l_j1j2*(m2 + m3))*sin(psi1)*psi1d, (l_j2g2*m2 + l_j2j3*m3)*sin(psi2)*psi2d, l_j3g3*m3*sin(psi3)*psi3d;
     1/2*(l_j1g1*m1 + l_j1j2*(m2 + m3))*cos(psi1)*psi1d, 1/2*(l_j1g1*m1 + l_j1j2*(m2 + m3))*sin(psi1)*psi1d, -1/2*(l_j1g1*m1 + l_j1j2*(m2 + m3))*(xd*cos(psi1)+yd*sin(psi1))+1/2*(l_j2g2*l_j1j2*m2+l_j1j2*l_j2j3*m3)*sin(psi1-psi2)*psi2d+1/2*l_j3g3*l_j1j2*m3*sin(psi1-psi3)*psi3d, (l_j2g2*l_j1j2*m2+l_j1j2*l_j2j3*m3)*sin(psi1-psi2)*(-1/2*psi1d+psi2d), l_j3g3*l_j1j2*m3*sin(psi1-psi3)*(-1/2*psi1d+psi3d);
     1/2*(l_j2g2*m2 + l_j2j3*m3)*cos(psi2)*psi2d, 1/2*(l_j2g2*m2 + l_j2j3*m3)*sin(psi2)*psi2d, (l_j2g2*l_j1j2*m2+l_j1j2*l_j2j3*m3)*sin(psi1-psi2)*(-psi1d+1/2*psi2d), -1/2*(l_j2g2*m2+l_j2j3*m3)*(xd*cos(psi2)+yd*sin(psi2))-1/2*(l_j2g2*l_j1j2*m2+l_j1j2*l_j2j3*m3)*sin(psi1-psi2)*psi1d+1/2*l_j3g3*l_j2j3*m3*sin(psi2-psi3)*psi3d, l_j3g3*l_j2j3*m3*sin(psi2-psi3)*(-1/2*psi2d+psi3d);
     1/2*l_j3g3*m3*cos(psi3)*psi3d, 1/2*l_j3g3*m3*sin(psi3)*psi3d, l_j3g3*l_j1j2*m3*sin(psi1-psi3)*(-psi1d+1/2*psi3d), l_j3g3*l_j2j3*m3*sin(psi2-psi3)*(-psi2d+1/2*psi3d), -1/2*l_j3g3*m3*(xd*cos(psi3)+yd*sin(psi3))-1/2*l_j3g3*l_j1j2*m3*sin(psi1-psi3)*psi1d-1/2*l_j3g3*l_j2j3*m3*sin(psi2-psi3)*psi2d;];

end

== matlab function time-domain-test/single-funky-sattyre-nonlinear-variable-crrc/M ==
  data: M output; q input
function M = calculate_M(q)

%%%%%%%%%%%%%%%%%%%%%%%%%%%%%%%%%%%%%%%%%%%%%%%%%%%%%%%%%%%%%%%%%%%%%%%%%%
% Parameter given
% M J L xg = mass, moment of inertia, length, cg location measured from rear joint

MM = [11.142, 7.651, 11.142]' * 1000; 
JJ = [143.57, 37.8, 143.57]' * 1000; 
LL = [11.4, 9.4, 11.4]';
XG = [5.538, 4.757, 11.4 - 5.538]';
XX = LL - XG;
%%%%%%%%%%%%%%%%%%%%%%%%%%%%%%%%%%%%%%%%%%%%%%%%%%%%%%%%%%%%%%%%%%%%%%%%%%
% Specify matrix dimensions in advance

P = zeros(6, 5); 
M = zeros(5, 5);
%%%%%%%%%%%%%%%%%%%%%%%%%%%%%%%%%%%%%%%%%%%%%%%%%%%%%%%%%%%%%%%%%%%%%%%%%%
% Rotation matrix

uu = zeros(2, 3); 
nn = zeros(2, 3); 
for i = 1:3
    c = cos(q(i + 2));
    s = sin(q(i + 2)); 
    uu(:, i)=[c, s]';
    nn(:, i)=[-s, c]';
end
%%%%%%%%%%%%%%%%%%%%%%%%%%%%%%%%%%%%%%%%%%%%%%%%%%%%%%%%%%%%%%%%%%%%%%%%%%
% Matrix generate

D1 = diag(kron(MM', [1 1]));    % 17
D2 = diag([0 0 JJ']);   % 18

P1 = kron(ones(3, 1), eye(2)); 
P2 = zeros(6, 3);
for i = 1:3
    for j = 1:3
        if i > j
            P2(2 * i - 1 : 2 * i, j) = -LL(j) * nn(:, j);
        elseif i == j
            P2(2 * i - 1 : 2 * i, j) = -XX(j) * nn(:, j);
        end
    end
end
P = [P1, P2];    % 15

M = P' * D1 * P + D2;

== matlab function time-domain-test/double-general-lineartyre-nonlinear-variable-matrix1/D ==
  data: D output
function D = calculate_D()

d1 = 10000;
d2 = 10000;

delta_kj = eye(3);
dj = [0, d1, d2, 0]';
D = zeros(5);

for k = 1:5
    for l = 1:5
        if k > 2 && l > 2
            if  l == k
                D(k, l) = (1 - delta_kj(1, k-2))*dj(k - 2) + (1 - delta_kj(3, k-2))*dj(k - 1);
            elseif l == k-1
                D(k, l) = -(1 - delta_kj(1, k-2))*dj(k - 2);
            elseif l == k+1
                D(k, l) = -(1 - delta_kj(3, k-2))*dj(k - 1);
            else
                D(k, l) = 0;
            end
        end
    end
end

end

== matlab function time-domain-test/double-general-lineartyre-nonlinear-variable-matrix1/M ==
  data: M output; q input
function M = calculate_M(q)

psi1 = q(3);
psi2 = q(4);
psi3 = q(5);

m1 = 11142;
m3 = 11142;
m2 = 7651; 
l_j1j2 = 11.4;
l_j2j3 = 9.4;
l_j1g1 = 5.862; 
l_j2g2 = 4.643; 
l_j3g3 = 5.538; 
iz1 = 143570; 
iz3 = 143570; 
iz2 = 37800;

l_kj = [l_j1g1, l_j1j2, l_j1j2;
             0, l_j2g2, l_j2j3;
             0,      0, l_j3g3;];
delta_kj = eye(3);
Jc = zeros(3, 5, 3);
for j = 1:3
    Jc(:, :, j) = [1, 0,  l_kj(1, j) * sin(psi1),  l_kj(2, j) * sin(psi2),  l_kj(3, j) * sin(psi3);
          0, 1, -l_kj(1, j) * cos(psi1), -l_kj(2, j) * cos(psi2), -l_kj(3, j) * cos(psi3);
          0, 0,          delta_kj(1, j),          delta_kj(2, j),          delta_kj(3, j);];
end

mj = [m1, m2, m3]';
izj = [iz1, iz2, iz3]';
Mj = zeros(3, 3, 3);
for j = 1:3
    Mj(:, :, j) = diag([mj(j), mj(j), izj(j)]);
end

M = zeros(5, 5);
for j = 1:3
    M = M + Jc(:, :, j)' * Mj(:, :, j) * Jc(:, :, j);
end

end

== matlab function time-domain-test/single-funky-sattyre-nonlinear-variable-crrc/dTdq ==
  data: q input; qd input; dTdq output
function dTdq = calculate_dTdq(q, qd)

%%%%%%%%%%%%%%%%%%%%%%%%%%%%%%%%%%%%%%%%%%%%%%%%%%%%%%%%%%%%%%%%%%%%%%%%%%
% Parameter given
% M J L xg = mass, moment of inertia, length, cg location measured from rear joint

MM = [11.142, 7.651, 11.142]' * 1000; 
JJ = [143.57, 37.8, 143.57]' * 1000; 
LL = [11.4, 9.4, 11.4]';
XG = [5.538, 4.757, 11.4 - 5.538]';
XX = LL - XG;
%%%%%%%%%%%%%%%%%%%%%%%%%%%%%%%%%%%%%%%%%%%%%%%%%%%%%%%%%%%%%%%%%%%%%%%%%%
% Specify matrix dimensions in advance

P = zeros(6, 5); 
R = zeros(6, 5); 
M = zeros(5, 5);
Xa = zeros(2, 8); 
Xj = zeros(2, 4); 
Xg = zeros(2, 3); 
%%%%%%%%%%%%%%%%%%%%%%%%%%%%%%%%%%%%%%%%%%%%%%%%%%%%%%%%%%%%%%%%%%%%%%%%%%
% Rotation matrix

uu = zeros(2, 3); 
nn = zeros(2, 3); 
for i = 1:3
    c = cos(q(i + 2));
    s = sin(q(i + 2)); 
    uu(:, i)=[c, s]';
    nn(:, i)=[-s, c]';
end
%%%%%%%%%%%%%%%%%%%%%%%%%%%%%%%%%%%%%%%%%%%%%%%%%%%%%%%%%%%%%%%%%%%%%%%%%%
% Matrix generate

D1 = diag(kron(MM', [1 1]));    % 17
D2 = diag([0 0 JJ']);   % 18

P1 = kron(ones(3, 1), eye(2)); 
P2 = zeros(6, 3);
for i = 1:3
    for j = 1:3
        if i > j
            P2(2 * i - 1 : 2 * i, j) = -LL(j) * nn(:, j);
        elseif i == j
            P2(2 * i - 1 : 2 * i, j) = -XX(j) * nn(:, j);
        end
    end
end
P = [P1, P2];    % 15

R1 = zeros(6, 2);
R2 = zeros(6, 3);
for i = 1:3
    for j = 1:3
        if i > j
            R2(2 * i - 1 : 2 * i, j) = LL(j) * uu(:, j);
        elseif i==j
            R2(2 * i - 1 : 2 * i, j) = XX(j) * uu(:, j);
        end
    end
end
R = [R1, R2];
%%%%%%%%%%%%%%%%%%%%%%%%%%%%%%%%%%%%%%%%%%%%%%%%%%%%%%%%%%%%%%%%%%%%%%%%%%
% calculate C 23

dTdq = zeros(5, 1); 
temp = qd' * P' * D1 * R;
dTdq = temp' .* qd;
%%%%%%%%%%%%%%%%%%%%%%%%%%%%%%%%%%%%%%%%%%%%%%%%%%%%%%%%%%%%%%%%%%%%%%%%%%
end

== matlab function time-domain-test/single-funky-sattyre-nonlinear-variable-crrc/generate qd ==
  data: M input; qd output; Mqd input
function qd = calqulate_qd(M, Mqd)
 
qd = M \ Mqd;

end

== matlab function time-domain-test/single-funky-sattyre-nonlinear-variable-crrc/origin_state ==
  data: M input; Mqd0 output; qd input
function Mqd0 = origin_state(M, qd)

Mqd0 = M * qd;

end

== matlab function time-domain-test/single-general-lineartyre-nonlinear-variable-crrc/C ==
  data: q input; qd input; C output
function C = calculate_C(q, qd)

% coefficient

m1 = 11142;
m3 = 11142;
m2 = 7651; 
l_j1j2 = 11.4;
l_j2j3 = 9.4;
l_j1g1 = 5.862; 
l_j2g2 = 4.643; 
l_j3g3 = 5.538; 

MM = [m1, m2, m3]';
LL = [l_j1j2, l_j2j3, l_j1j2]';
XX = [l_j1g1, l_j2g2, l_j3g3]';

% Rotation matrix

uu = zeros(2, 3);
nn = zeros(2, 3);
for i = 1:3
    uu(:, i)=[cos(q(i + 2)), sin(q(i + 2))]';
    nn(:, i)=[-sin(q(i + 2)), cos(q(i + 2))]';
end

% Matrix generate
% Specify matrix dimensions in advance

D1 = diag(kron(MM', [1 1]));

P1 = kron(ones(3, 1), eye(2));
P2 = zeros(6, 3);
for i = 1:3
    for j = 1:3
        if i > j
            P2(2 * i - 1 : 2 * i, j) = -LL(j) * nn(:, j);
        elseif i == j
            P2(2 * i - 1 : 2 * i, j) = -XX(j) * nn(:, j);
        else
            P2(2 * i - 1 : 2 * i, j) = 0;
        end
    end
end
P = [P1, P2];

R1 = zeros(6, 2);
R2 = zeros(6, 3);
for i = 1:3
    for j = 1:3
        if i > j
            R2(2 * i - 1 : 2 * i, j) = LL(j) * uu(:, j);
        elseif i==j
            R2(2 * i - 1 : 2 * i, j) = XX(j) * uu(:, j);
        else
            R2(2 * i - 1 : 2 * i, j) = 0;
        end
    end
end
R = [R1, R2];

dTdq = (qd' * P' * D1 * R)' .* qd;

Pd1 = zeros(6, 2);
Pd2 = zeros(6, 3);
for i = 1:3
    for j = 1:3
        if i > j
            Pd2(2 * i - 1 : 2 * i, j) = LL(j) * uu(:, j) * qd(j + 2);
        elseif i==j
            Pd2(2 * i - 1 : 2 * i, j) = XX(j) * uu(:, j) * qd(j + 2);
        else
            Pd2(2 * i - 1 : 2 * i, j) = 0;
        end
    end
end
Pd = [Pd1, Pd2];
Md = Pd'*D1*P + P'*D1*Pd;

C = Md*qd - dTdq;
end

== matlab function time-domain-test/single-general-lineartyre-nonlinear-variable-crrc/M ==
  data: M output; q input
function M = calculate_M(q)

% coefficient

m1 = 11142;
m3 = 11142;
m2 = 7651; 
l_j1j2 = 11.4;
l_j2j3 = 9.4;
l_j1g1 = 5.862; 
l_j2g2 = 4.643; 
l_j3g3 = 5.538; 
iz1 = 143570; 
iz3 = 143570; 
iz2 = 37800;
MM = [m1, m2, m3]';
JJ = [iz1, iz2, iz3]';
LL = [l_j1j2, l_j2j3, l_j1j2]';
XX = [l_j1g1, l_j2g2, l_j3g3]';

% Rotation matrix

uu = zeros(2, 3);
nn = zeros(2, 3);
for i = 1:3
    uu(:, i)=[cos(q(i + 2)), sin(q(i + 2))]';
    nn(:, i)=[-sin(q(i + 2)), cos(q(i + 2))]';
end

% Matrix generate
% Specify matrix dimensions in advance

D1 = diag(kron(MM', [1 1]));
D2 = diag([0 0 JJ']);

P1 = kron(ones(3, 1), eye(2));
P2 = zeros(6, 3);
for i = 1:3
    for j = 1:3
        if i > j
            P2(2 * i - 1 : 2 * i, j) = -LL(j) * nn(:, j);
        elseif i == j
            P2(2 * i - 1 : 2 * i, j) = -XX(j) * nn(:, j);
        else
            P2(2 * i - 1 : 2 * i, j) = 0;
        end
    end
end
P = [P1, P2];

M = P' * D1 * P + D2;

== matlab function time-domain-test/double-general-lineartyre-nonlinear-variable-matrix1/Tau_tire ==
  data: q input; qd input; delta input; Fx input; Tau_tire output; Alpha output
function [Tau_tire, Alpha] = calculate_Tau_tire(q, qd, delta, Fx)

% coefficient

l_j1j2 = 11.4;
l_j2j3 = 9.4;
l_j1a1 = 2.5;
l_j1a2 = 4;
l_j1a3 = 9.9;
l_j2a4 = 1.5;
l_j2a5 = 7.9;
l_j3a6 = 1.5;
l_j3a7 = 7.4;
l_j3a8 = 8.9;
h11 = 0.9625;
h12 = 0.9625;
h13 = 0.98;
h21 = 0.98; 
h22 = 0.98;
h31 = 0.98;
h32 = 0.9625;
h33 = 0.9625;
ca1 = 3065 * 180 / pi;
ca2 = 3065 * 180 / pi;
ca3 = 3065 * 180 / pi;
ca4 = 3065 * 180 / pi;
ca5 = 3065 * 180 / pi;
ca6 = 3065 * 180 / pi;
ca7 = 3065 * 180 / pi;
ca8 = 3065 * 180 / pi;

x = q(1);
y = q(2);
psi1 = q(3);
psi2 = q(4);
psi3 = q(5);
xd = qd(1);
yd = qd(2);
psi1d = qd(3);
psi2d = qd(4);
psi3d = qd(5);

psij = [psi1, psi2, psi3]';
Rot_w2v = zeros(2, 2, 3);
for i = 1:3
    Rot_w2v(:, :, i) = [cos(psij(i)), -sin(psij(i));
                        sin(psij(i)), cos(psij(i));];
end

Rot_v2t = zeros(2, 2, 8);
for i = 1:8
    Rot_v2t(:, :, i) = [cos(delta(i)), -sin(delta(i));
                        sin(delta(i)), cos(delta(i));];
end

xj = zeros(3, 1);
yj = zeros(3, 1);
xj(1) = x;
yj(1) = y;
xj(2) = x - l_j1j2*cos(psi1);
yj(2) = y - l_j1j2*sin(psi1);
xj(3) = x - l_j1j2*cos(psi1) - l_j2j3*cos(psi2);
yj(3) = y - l_j1j2*sin(psi1) - l_j2j3*sin(psi2);

u = zeros(2, 3);
n = zeros(2, 3);
for i = 1:3
    u(:, i)=[cos(q(i + 2)), sin(q(i + 2))]';
    n(:, i)=[-sin(q(i + 2)), cos(q(i + 2))]';
end

IU = [1, 1, 1, 2, 2, 3, 3, 3]';
l_ja = [l_j1a1, l_j1a2, l_j1a3, l_j2a4, l_j2a5, l_j3a6, l_j3a7, l_j3a8]';
ha = [h11, h12, h13, h21, h22, h31, h32, h33]';

L_long1 = [cos(psi1), cos(psi1), cos(psi1), cos(psi2), cos(psi2), cos(psi3), cos(psi3), cos(psi3);
           sin(psi1), sin(psi1), sin(psi1), sin(psi2), sin(psi2), sin(psi3), sin(psi3), sin(psi3);
           -h11, -h12, -h13, l_j1j2*sin(psi1-psi2), l_j1j2*sin(psi1-psi2), l_j1j2*sin(psi1-psi3), l_j1j2*sin(psi1-psi3), l_j1j2*sin(psi1-psi3);
           0, 0, 0, -h21, -h22, l_j2j3*sin(psi2-psi3), l_j2j3*sin(psi2-psi3), l_j2j3*sin(psi2-psi3);
           0, 0, 0, 0, 0, -h31, -h32, -h33;];

L_long2 = [cos(psi1), cos(psi1), cos(psi1), cos(psi2), cos(psi2), cos(psi3), cos(psi3), cos(psi3);
           sin(psi1), sin(psi1), sin(psi1), sin(psi2), sin(psi2), sin(psi3), sin(psi3), sin(psi3);
           h11, h12, h13, l_j1j2*sin(psi1-psi2), l_j1j2*sin(psi1-psi2), l_j1j2*sin(psi1-psi3), l_j1j2*sin(psi1-psi3), l_j1j2*sin(psi1-psi3);
           0, 0, 0, h21, h22, l_j2j3*sin(psi2-psi3), l_j2j3*sin(psi2-psi3), l_j2j3*sin(psi2-psi3);
           0, 0, 0, 0, 0, h31, h32, h33;];

L_lat1 = [-sin(psi1), -sin(psi1), -sin(psi1), -sin(psi2), -sin(psi2), -sin(psi3), -sin(psi3), -sin(psi3);
          cos(psi1), cos(psi1), cos(psi1), cos(psi2), cos(psi2), cos(psi3), cos(psi3), cos(psi3);
          -l_j1a1, -l_j1a2, -l_j1a3, -l_j1j2*cos(psi1-psi2), -l_j1j2*cos(psi1-psi2), -l_j1j2*cos(psi1-psi3), -l_j1j2*cos(psi1-psi3), -l_j1j2*cos(psi1-psi3);
          0, 0, 0, -l_j2a4, -l_j2a5, -l_j2j3*cos(psi2-psi3), -l_j2j3*cos(psi2-psi3), -l_j2j3*cos(psi2-psi3);
          0, 0, 0, 0, 0, -l_j3a6, -l_j3a7, -l_j3a8;];

L_lat2 = [-sin(psi1), -sin(psi1), -sin(psi1), -sin(psi2), -sin(psi2), -sin(psi3), -sin(psi3), -sin(psi3);
          cos(psi1), cos(psi1), cos(psi1), cos(psi2), cos(psi2), cos(psi3), cos(psi3), cos(psi3);
          -l_j1a1, -l_j1a2, -l_j1a3, -l_j1j2*cos(psi1-psi2), -l_j1j2*cos(psi1-psi2), -l_j1j2*cos(psi1-psi3), -l_j1j2*cos(psi1-psi3), -l_j1j2*cos(psi1-psi3);
          0, 0, 0, -l_j2a4, -l_j2a5, -l_j2j3*cos(psi2-psi3), -l_j2j3*cos(psi2-psi3), -l_j2j3*cos(psi2-psi3);
          0, 0, 0, 0, 0, -l_j3a6, -l_j3a7, -l_j3a8;];

Delta_c = zeros(8, 8);
Delta_s = zeros(8, 8);
for i = 1:8
    Delta_c(i, i) = cos(delta(i));
    Delta_s(i, i) = sin(delta(i));
end

vxj = zeros(3, 1);
vyj = zeros(3, 1);
vxj(1) = xd;
vyj(1) = yd;
vxj(2) = xd + l_j1j2*sin(psi1)*psi1d;
vyj(2) = yd - l_j1j2*cos(psi1)*psi1d;
vxj(3) = xd + l_j1j2*sin(psi1)*psi1d + l_j2j3*sin(psi2)*psi2d;
vyj(3) = yd - l_j1j2*cos(psi1)*psi1d - l_j2j3*cos(psi2)*psi2d;
va1 = zeros(2, 8);
va2 = zeros(2, 8);
psidj = [psi1d, psi2d, psi3d]';
for i = 1:8
    va1(:, i) = [vxj(IU(i)); vyj(IU(i))] - n(:, IU(i))*l_ja(i)*psidj(IU(i)) + (-1)*u(:, IU(i))*ha(i)*psidj(IU(i));
    va2(:, i) = [vxj(IU(i)); vyj(IU(i))] - n(:, IU(i))*l_ja(i)*psidj(IU(i)) + u(:, IU(i))*ha(i)*psidj(IU(i));
end

va1_v = zeros(2, 8);
va2_v = zeros(2, 8);
for i = 1:8
    va1_v(:, i) = inv(Rot_w2v(:, :, IU(i)))*va1(:, i);
    va2_v(:, i) = inv(Rot_w2v(:, :, IU(i)))*va2(:, i);
end

beta1 = zeros(8, 1);
beta2 = zeros(8, 1);
for i = 1:8
    beta1(i) = atan2(va1_v(2, i), va1_v(1, i));
    beta2(i) = atan2(va2_v(2, i), va2_v(1, i));
end

ca = [ca1, ca2, ca3, ca4, ca5, ca6, ca7, ca8]';
Ca = diag(ca);

Tau_tire = L_long1 * (Delta_c * Fx / 2 - Delta_s * Ca * (delta - beta1)) ...
         + L_long2 * (Delta_c * Fx / 2 - Delta_s * Ca * (delta - beta2)) ...
         + L_lat1 * (Delta_s * Fx / 2 + Delta_c * Ca * (delta - beta1)) ...
         + L_lat2 * (Delta_s * Fx / 2 + Delta_c * Ca * (delta - beta2));

beta = (beta1 + beta2) / 2;
Alpha = delta - beta;

end

== matlab function time-domain-test/single-general-lineartyre-nonlinear-variable-crrc/Q ==
  data: q input; qd input; delta input; Fx input; Q output; Alpha output
function [Q, Alpha] = calculate_Q(q, qd, delta, Fx)

% coefficient

l_j1j2 = 11.4;
l_j2j3 = 9.4;
l_j1a1 = 2.5;
l_j1a2 = 4;
l_j1a3 = 9.9;
l_j2a4 = 1.5;
l_j2a5 = 7.9;
l_j3a6 = 1.5;
l_j3a7 = 7.4;
l_j3a8 = 8.9;

LL = [l_j1j2, l_j2j3, l_j1j2]';
JA = [l_j1a1, l_j1a2, l_j1a3, l_j2a4, l_j2a5, l_j3a6, l_j3a7, l_j3a8]';
XA = [l_j1j2, l_j1j2, l_j1j2, l_j2j3, l_j2j3, l_j1j2, l_j1j2, l_j1j2]' - JA;
IU = [1, 1, 1, 2, 2, 3, 3, 3]';

Ca = [3065 * 180 / pi, 3065 * 180 / pi, 3065 * 180 / pi, 3065 * 180 / pi, 3065 * 180 / pi, 3065 * 180 / pi, 3065 * 180 / pi, 3065 * 180 / pi]';

uu = zeros(2, 3);
nn = zeros(2, 3);
for i = 1:3
    uu(:, i)=[cos(q(i + 2)), sin(q(i + 2))]';
    nn(:, i)=[-sin(q(i + 2)), cos(q(i + 2))]';
end

Va = zeros(2, 8);      % axle velocities in globals
Vj = zeros(2, 4);      % joint velocities in globals
Va_v = Va;             % axle velocities in locals

xd = qd(1);
yd = qd(2);
Vj(:, 1) = [xd, yd]';
for i = 1:3
    Vj(:, i+1) = Vj(:, i) - qd(i + 2) * LL(i) * nn(:, i);
end

for i = 1:8
    Va(:, i) = Vj(:, IU(i) + 1) + qd(IU(i) + 2) * XA(i) * nn(:, IU(i));
    Vax_v = dot(Va(:, i), uu(:, IU(i)));
    Vay_v = dot(Va(:, i), nn(:, IU(i)));
    Va_v(:, i) = [Vax_v; Vay_v];
end

Fy = zeros(8, 1); 
Alpha = zeros(8, 1); 

for i = 1:8
    vx = Va_v(1, i) * cos(delta(i)) + Va_v(2, i) * sin(delta(i));
    vy = -Va_v(1, i) * sin(delta(i)) + Va_v(2, i) * cos(delta(i));
    alpha = atan2(vy, vx);
    Alpha(i) = alpha;
    Fy(i) = -abs(Ca(i) * alpha) * sign(vy);
end

J = zeros(2, 5);
Q = zeros(5, 1);

ua = zeros(2, 8);
na = zeros(2, 8);
for i = 1:8
    ua(:, i)=[cos(q(IU(i) + 2) + delta(i)), sin(q(IU(i) + 2) + delta(i))]';
    na(:, i)=[-sin(q(IU(i) + 2) + delta(i)), cos(q(IU(i) + 2) + delta(i))]';
end

for i = 1:8
    Fa = [Fx(i); Fy(i)];
    iu = IU(i); 
    u = ua(:, i);
    n = na(:, i); 

    for j = 1:5
        J(:, j) = [0; 0];
    end
    J(1, 1) = 1; 
    J(2, 2) = 1;

    for j = 1:iu
        if j < iu
            J(:, j + 2) = -LL(j) * nn(:, j);
        else
            J(:, j + 2) = -(LL(j) - XA(i)) * nn(:, j);
        end
    end
    Q = Q + J' * [u n] * Fa;
end

end

== matlab function time-domain-test/proc/MatMaker ==
  data: Va output; Vaa output; Vj output; q input; qd input; Vg output; PARSu input; PARSa input; Vgg output
function [Va,Vaa,Vj,Vg,Vgg] =Vmaker(q,qd,PARSu,PARSa)


%%%%%%%%%%%%%%%%%%%%%%%%%%%%%%%%%%%%%%%%%%%%%%%%%%%%%%%%%%%%%%%%%%%%%%%%%

Va=zeros(2,8); % (2,Na) - axle velocities in globals
Vj=zeros(2,4); % (2,Nu+1) - joint velocities in globals
Vg=zeros(2,3); % (2,Nu) - CG velocities in globals
%%%%%%%%%%%%%%%%%%%%%%%%%%%%%%%%%%%%%%%%%%%%%%%%%%%%%%%%%%%%%%%%%%%%%%%%%%
Vaa=Va; % axle velocities in locals
Vgg=Vg; % CG velocities in locals

% actual dimensions
Nu=size(PARSu,1);
Na=size(PARSa,1);

LL=PARSu(:,3);
XG=PARSu(:,4);
XX=LL-XG;

uu=zeros(2,Nu); 
nn=zeros(2,Nu);
for i=1:Nu
    c=cos(q(i+2));s=sin(q(i+2));
    uu(:,i)=[c,s]';
    nn(:,i)=[-s,c]';
end


Vj(:,1)=[qd(1),qd(2)]';
for i=1:Nu
    Vj(:,i+1)=Vj(:,i)-qd(i+2)*LL(i)*nn(:,i);%negative sign since working backwards
    Vg(:,i)=Vj(:,i)-qd(i+2)*XX(i)*nn(:,i);
    Vgx=dot(Vg(:,i),uu(:,i));Vgy=dot(Vg(:,i),nn(:,i));
    Vgg(:,i)=[Vgx;Vgy];
end

%velocities at axles 
for i=1:Na
    xa=PARSa(i,1);
    k=PARSa(i,2);
    Va(:,i)=Vj(:,k+1)+qd(k+2)*xa*nn(:,k);
    Vax=dot(Va(:,i),uu(:,k));Vay=dot(Va(:,i),nn(:,k));
    Vaa(:,i)=[Vax;Vay];
end

== matlab function time-domain-test/single-funky-sattyre-nonlinear-variable-crrc/V_tyre ==
  data: q input; Vaa output; qd input
function Vaa = calculate_v_tyre(q, qd)

%%%%%%%%%%%%%%%%%%%%%%%%%%%%%%%%%%%%%%%%%%%%%%%%%%%%%%%%%%%%%%%%%%%%%%%%%
Va = zeros(2, 8); % axle velocities in globals
Vj = zeros(2, 4); % joint velocities in globals
Vaa = Va; % axle velocities in locals
%%%%%%%%%%%%%%%%%%%%%%%%%%%%%%%%%%%%%%%%%%%%%%%%%%%%%%%%%%%%%%%%%%%%%%%%%%
% Parameter given
% M J L xg = mass, moment of inertia, length, cg location measured from rear joint

LL = [11.4, 9.4, 11.4]';
XG = [5.538, 4.757, 11.4 - 5.538]';
XA = [8.9, 7.4, 1.5, 7.9, 1.5, 9.9, 4.0, 2.5]';
KK = [1, 1, 1, 2, 2, 3, 3, 3]';
%%%%%%%%%%%%%%%%%%%%%%%%%%%%%%%%%%%%%%%%%%%%%%%%%%%%%%%%%%%%%%%%%%%%%%%%%%
% Rotation matrix

uu = zeros(2, 3); 
nn = zeros(2, 3); 
for i = 1:3
    c = cos(q(i + 2));
    s = sin(q(i + 2)); 
    uu(:, i) = [c, s]';
    nn(:, i) = [-s, c]';
end
%%%%%%%%%%%%%%%%%%%%%%%%%%%%%%%%%%%%%%%%%%%%%%%%%%%%%%%%%%%%%%%%%%%%%%%%%%
% % from first unit cg to first virtual joint
% 
% l = 11.4;
% b1 = 5.538;
% 
% q = zeros(5,1);
% q(1) = q(1) + (l - b1) * cos(q(3));
% q(2) = q(2) + (l - b1) * sin(q(3));
% 
% qd = zeros(5,1);
% qd(1) = qd(1) + (l - b1) * qd(3) * sin(q(3));
% qd(2) = qd(2) - (l - b1) * qd(3) * cos(q(3));
%%%%%%%%%%%%%%%%%%%%%%%%%%%%%%%%%%%%%%%%%%%%%%%%%%%%%%%%%%%%%%%%%%%%%%%%%%
% calculate v_tyre

Vj(:, 1) = [qd(1), qd(2)]';

for i = 1:3
    Vj(:, i+1) = Vj(:, i) - qd(i + 2) * LL(i) * nn(:, i);
end

for i = 1:8
    Va(:, i) = Vj(:, KK(i) + 1) + qd(KK(i) + 2) * XA(i) * nn(:, KK(i));
    Vax = dot(Va(:, i), uu(:, KK(i)));
    Vay = dot(Va(:, i), nn(:, KK(i)));
    Vaa(:, i) = [Vax; Vay];
end
%%%%%%%%%%%%%%%%%%%%%%%%%%%%%%%%%%%%%%%%%%%%%%%%%%%%%%%%%%%%%%%%%%%%%%%%%%

== matlab function time-domain-test/single-general-lineartyre-nonlinear-variable-crrc/qdd ==
  data: M input; C input; Q input; qdd output
function qdd = calculate_qdd(M, C, Q)

qdd = inv(M)*(Q - C);

end
